simulink library "platooning_custom_blocks"  (R2018b)
settings: Solver=VariableStepAuto  StartTime=0.0  StopTime=10.0  RelTol=1e-3
undefined symbols (not defined in the file): AccPdl_pdlbpt, AccPdl_spdbpt, AccPdl_trqMap, adj_motEffMap, BETModel, BrkPdl_brkTrq, BrkPdl_pdlbpt, Cd_Map, Cd_Map_T2, CT_accPdl_pdlbpt, CT_accPdl_spdbpt, CT_accPdl_trqMap, CT_brkPdl_brkTrq, CT_brkPdl_pdlbpt, CTModel, d_11, d_22, DiscIntNeverNeededParam, init_veh_spd_mps, max_Cd_frac, min_Cd_frac, motSpdVec, motTrqVec, msk_init_pos_m, msk_mot_cont_trq, msk_mot_num, msk_mot_spd_bpt, N_OptResults, sim_t_step, simDrv, SPHETModel, t_step
libraries: simulink x19, $bdroot x16, dspstat3 x2, custom_func x1
(part 1 of 5)
settings Model: Creator=Aman-Home  LastModifiedBy=Aman-Home

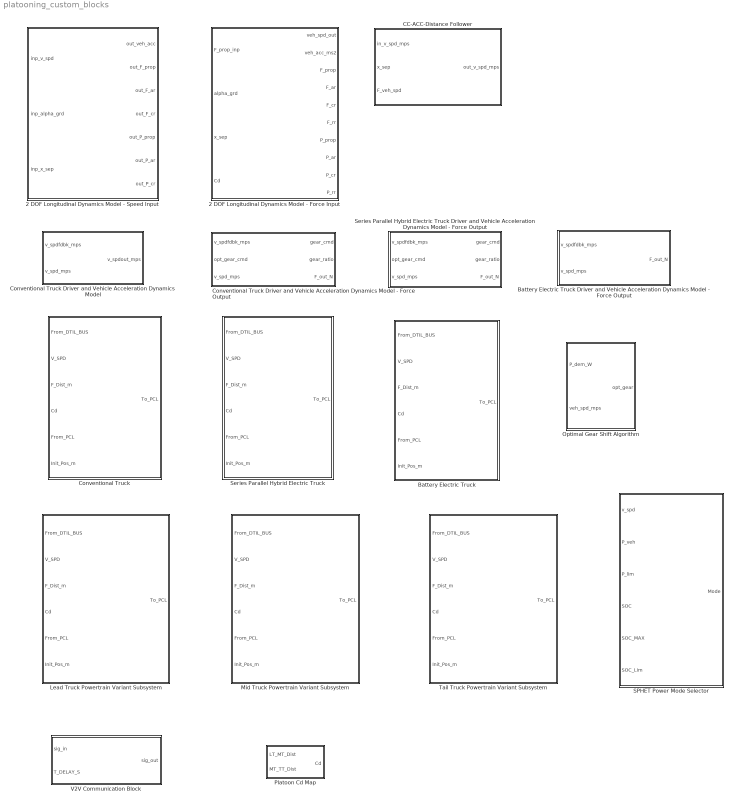
== system platooning_custom_blocks ==
  2 DOF Longitudinal Dynamics Model - Force Input : Subsystem  mask{msk_mass=CTModel.veh_mass_kg, msk_Af=CTModel.Af_m2, msk_Cd=CTModel.Cd_avg * ones([3 1]), msk_Cd_bpt=[5;10;15], msk_r_tire=CTModel.ld_tire_rad_m, msk_v_init=init_veh_spd_mps, msk_roadType=Smooth Concrete, msk_rho_air=1.227, msk_tstep=sim_t_step}
      mask prompts: msk_mass "Vehicle Mass [kg]:"; msk_Af "Vehicle Frontal Area [m^2]:"; msk_Cd "Vehicle Coefficient of Drag, Data Vector [n-by-1] (-):"; msk_Cd_bpt "Vehicle Coefficient of Drag, Breakpoint Vector [n-by-1] (meters):"; msk_r_tire "Vehicle Tire Radius [m]:"; msk_v_init "Vehicle Initial Speed [m/s]:"; msk_roadType "Road Type:"; msk_rho_air "Air density [kg/m^3]:"; msk_tstep "Simulation time step [s]:"
      mask init:
      | switch msk_roadType
      |     case 'Smooth Concrete'
      |         msk_roadType = 0;
      |     case 'Worn Concrete'
      |         msk_roadType = 1;
      |     case 'Hot Blacktop'
      |         msk_roadType = 2;
      | end
      mask TypeOptions msk_roadType: Smooth Concrete | Worn Concrete | Hot Blacktop
      mask DialogControl Container3 Prompt: Vehicle Parameters
      mask DialogControl Container6 Prompt: Road Parameters
      mask DialogControl Container7 Prompt: Environmental Parameters
      mask DialogControl Container9 Prompt: Simulation Parameters
  2 DOF Longitudinal Dynamics Model - Speed Input : Subsystem  mask{msk_mass=35380, msk_Af=4.5, msk_Cd=[0.3;0.2;0.1], msk_Cd_bpt=[5;10;15], msk_r_tire=0.5435, msk_roadType=Smooth Concrete, msk_rho_air=1.227, msk_tstep=t_step}
      mask prompts: msk_mass "Vehicle Mass [kg]:"; msk_Af "Vehicle Frontal Area [m^2]:"; msk_Cd "Vehicle Coefficient of Drag, Data Vector [n-by-1] (-):"; msk_Cd_bpt "Vehicle Coefficient of Drag, Breakpoint Vector [n-by-1] (meters):"; msk_r_tire "Vehicle Tire Radius [m]:"; msk_roadType "Road Type:"; msk_rho_air "Air density [kg/m^3]:"; msk_tstep "Simulation time step [s]:"
      mask init:
      | switch msk_roadType
      |     case 'Smooth Concrete'
      |         msk_roadType = 0;
      |     case 'Worn Concrete'
      |         msk_roadType = 1;
      |     case 'Hot Blacktop'
      |         msk_roadType = 2;
      | end
      mask TypeOptions msk_roadType: Smooth Concrete | Worn Concrete | Hot Blacktop
      mask DialogControl DescGroupVar Prompt: Description
      mask DialogControl DescTextVar Prompt: 2 DOF longitudinal vehicle dynamics model parameter settings.
      mask DialogControl Container3 Prompt: Vehicle Parameters
      mask DialogControl Container4 Prompt: Road Parameters
      mask DialogControl Container5 Prompt: Environment Parameters
      mask DialogControl Container6 Prompt: Simulation Parameters
  Battery Electric Truck : Subsystem  VariantControl=TT.Type == 3
  Battery Electric Truck Driver and Vehicle Acceleration Dynamics Model - Force Output : Subsystem  mask{msk_Kp=0.1, msk_Ki=0.001, msk_t_step=sim_t_step, msk_mtr_cont_trq=BETModel.cont_mtr_trq_map, msk_mtr_pk_trq=BETModel.peak_mtr_trq_map, msk_spd_bpt=BETModel.cont_mtr_trq_spdbpt, msk_gear_ratio=BETModel.gear_ratio, msk_num_motors=4, msk_acc_trqmap=AccPdl_trqMap, msk_acc_spdbpt=AccPdl_spdbpt, msk_acc_pdlbpt=AccPdl_pdlbpt, msk_brk_trq=BrkPdl_brkTrq, msk_brk_pdlbpt=BrkPdl_pdlbpt, msk_mass=BETModel.veh_mass_kg, msk_damp_acc=800, msk_damp_brk=0.1, msk_tire_radius=BETModel.ld_tire_rad_m, msk_brk_whl_num=10}
      mask prompts: msk_Kp "PI Control - Proportional Gain [Kp]:"; msk_Ki "PI Control - Integral Gain [Ki]:"; msk_t_step "Simulation time step [s]:"; msk_mtr_cont_trq "Motor Continuous Torque Vector []:"; msk_mtr_pk_trq "Motor Peak Torque Vector []:"; msk_spd_bpt "Motor Speed bpt []:"; msk_gear_ratio "Motor Gear Ratio []:"; msk_num_motors "Number of motors []:"; msk_acc_trqmap "Acceleration torque map:"; msk_acc_spdbpt "Acceleration torque map - speed breakpoint vector:"; msk_acc_pdlbpt "Acceleration torque map - pedal breakpoint vector:"; msk_brk_trq "Braking torque vector:"; msk_brk_pdlbpt "Braking torque - pedal breakpoint vector:"; msk_mass "Vehicle mass [kg]:"; msk_damp_acc "Vehicle system damping - acceleration [ms^-2]:"; msk_damp_brk "Vehicle system damping - braking [ms^-2]:"; msk_tire_radius "Vehicle tire radius [m]:"; msk_brk_whl_num "Number of Wheels with braking [-]:"
      mask DialogControl DescGroupVar Prompt: Driver Model Settings
      mask DialogControl DescTextVar Prompt: Enter parameters values and input data for the driver model.
      mask DialogControl Container3 Prompt: Motor Parameters
      mask DialogControl Container4 Prompt: Pedal Maps
      mask DialogControl Container5 Prompt: Vehicle Parameters
  CC-ACC-Distance Follower : Subsystem  mask{msk_cc_mode=Disabled, msk_cc_setspd=25, msk_cc_time=100, msk_ACC_Kp=0.5, msk_ACC_Ki=0.01, msk_ACC_Kd=0, msk_ACC_setdist_init=70, msk_platoon_time=200, msk_ACC_setdist_final=15}
      mask prompts: msk_cc_mode "Select the controller mode:"; msk_cc_setspd "Cruise Control Set Speed:"; msk_cc_time "Cruise Control Activation Time [s]:"; msk_ACC_Kp "ACC - Distance Control, Kp:"; msk_ACC_Ki "ACC - Distance Control, Ki:"; msk_ACC_Kd "ACC - Distance Control, Kd:"; msk_ACC_setdist_init "ACC - Pre-Platoon Distance Setting [m]:"; msk_platoon_time "ACC - Platooning Start Time [s]:"; msk_ACC_setdist_final "ACC - Platoon Distance Setting [m]:"
      mask init:
      | switch msk_cc_mode
      |     case 'Disabled'
      |         msk_cc_mode = 0;
      |     case 'Activate - Cruise Control'
      |         msk_cc_mode = 1;
      |     case 'Activate - Adaptive Cruise Control'
      |         msk_cc_mode = 2;
      |     case 'Activate - Distance Following'
      |         msk_cc_mode = 3;
      | end
      mask TypeOptions msk_cc_mode: Disabled | Activate - Cruise Control | Activate - Adaptive Cruise Control | Activate - Distance Following
      mask Callback msk_cc_mode:
      | % Get the mask parameter values. This is a cell
      | %   array of character vectors.
      | maskStr = get_param(gcb,'msk_cc_mode');
      | 
      | % The pop-up menu is the first mask parameter.
      | %   Check the value selected in the pop-up
      | if strcmp(maskStr(1),'A') && strcmp(maskStr(12),'C')    % Activated - Cruise Control
      | 
      |     % Set the visibility of both parameters on when
      |     %   User-defined is selected in the pop-up.
      |     set_param(gcb,'MaskVisibilities',{'on';'on';'on';'off';'off';'off';'off';'off';'off'})
      | 
      | elseif strcmp(maskStr(1),'A') && strcmp(maskStr(12),'A')    % Activated - Adaptive Cruise Control
      | 
      |     % Turn off the visibility of the Value field
      |     %   when User-defined is not selected.
      | 
      |     set_param(gcb,'MaskVisibilities',{'on';'on';'on';'on';'on';'on';'on';'on';'on'})
      | 
      | elseif strcmp(maskStr(1),'A') && strcmp(maskStr(12),'D')    % Activated - Distance Following
      | 
      |     set_param(gcb,'MaskVisibilities',{'on';'on';'on';'on';'on';'on';'on';'on';'on'})
      | 
      | else
      | 
      |      set_param(gcb,'MaskVisibilities',{'on';'off';'off';'off';'off';'off';'off';'off';'off'})
      | 
      |     % Set the character vector in the Values field equal to the
      |     % character vector selected in the Gain pop-up menu.
      | 
      |     %maskStr{2}=maskStr{1};
      |     %set_param(gcb,'t_shutfault',inf);
      | end
      mask DialogControl DescGroupVar Prompt: Autonomous Speed Controller
      mask DialogControl DescTextVar Prompt: This block is used to enable and disable Cruise Control (CC), Adaptive Cruise Control (ACC) and Distance Following (DF) algorithms.
  Conventional Truck : Subsystem  VariantControl=LT.Type == 1
  Conventional Truck Driver and Vehicle Acceleration Dynamics Model : Subsystem  mask{msk_Kp=0.0075, msk_Ki=0.005, msk_t_step=t_step, msk_gear_ratio_vec=[14.43,11.05,8.44,6.46,4.95,3.79,2.91,2.23,1.70], msk_gearShft_UL=[3, 5, 10, 14, 18, 22, 26, 32, 45], msk_gearShft_LL=[0, 2, 4, 8, 12, 16, 20, 24, 30], msk_gearInit=1, msk_acc_trqmap=CT_accPdl_trqMap, msk_acc_spdbpt=CT_accPdl_spdbpt, msk_acc_pdlbpt=CT_accPdl_pdlbpt, msk_brk_trq=CT_brkPdl_brkTrq, msk_brk_pdlbpt=CT_brkPdl_pdlbpt, msk_mass=35000, msk_damp_acc=800, msk_damp_brk=0.1, msk_fd_ratio=2.8, msk_tire_radius=0.5456, msk_max_trq=2100, msk_brk_whl_num=10}
      mask prompts: msk_Kp "PI Control - Proportional Gain [Kp]:"; msk_Ki "PI Control - Integral Gain [Ki]:"; msk_t_step "Simulation time step [s]:"; msk_gear_ratio_vec "Gear ratio vector []:"; msk_gearShft_UL "Gear shift speed - Upper Limit vector []:"; msk_gearShft_LL "Gear shift speed - Lower Limit vector []:"; msk_gearInit "Initial Gear (non-zero):"; msk_acc_trqmap "Acceleration torque map:"; msk_acc_spdbpt "Acceleration torque map - speed breakpoint vector:"; msk_acc_pdlbpt "Acceleration torque map - pedal breakpoint vector:"; msk_brk_trq "Braking torque vector:"; msk_brk_pdlbpt "Braking torque - pedal breakpoint vector:"; msk_mass "Vehicle mass [kg]:"; msk_damp_acc "Vehicle system damping - acceleration [ms^-2]:"; msk_damp_brk "Vehicle system damping - braking [ms^-2]:"; msk_fd_ratio "Vehicle final drive ratio []:"; msk_tire_radius "Vehicle tire radius [m]:"; msk_max_trq "Maximum Engine Torque [Nm]:"; msk_brk_whl_num "Number of Wheels with braking [-]:"
      mask DialogControl DescGroupVar Prompt: Driver Model Settings
      mask DialogControl DescTextVar Prompt: Enter parameters values and input data for the driver model.
      mask DialogControl Container3 Prompt: Gear Shift Parameters
      mask DialogControl Container4 Prompt: Pedal Maps
      mask DialogControl Container5 Prompt: Vehicle Parameters
  Conventional Truck Driver and Vehicle Acceleration Dynamics Model - Force Output : Subsystem  mask{msk_Kp=0.1, msk_Ki=0.001, msk_t_step=sim_t_step, msk_gear_ratio_vec=CTModel.gear_ratios, msk_gearShft_UL=[3, 5, 9, 13, 17, 21, 25, 29, 33, 45], msk_gearShft_LL=[0, 2, 4, 8, 12, 16, 20, 24, 28, 32], msk_gearInit=1, msk_acc_trqmap=AccPdl_trqMap, msk_acc_spdbpt=AccPdl_spdbpt, msk_acc_pdlbpt=AccPdl_pdlbpt, msk_brk_trq=BrkPdl_brkTrq, msk_brk_pdlbpt=BrkPdl_pdlbpt, msk_mass=CTModel.veh_mass_kg, msk_damp_acc=800, msk_damp_brk=0.1, msk_fd_ratio=CTModel.fd_ratio, msk_tire_radius=CTModel.ld_tire_rad_m, msk_max_trq=max(CTModel.peak_eng_trq_map), msk_brk_whl_num=10}
      mask prompts: msk_Kp "PI Control - Proportional Gain [Kp]:"; msk_Ki "PI Control - Integral Gain [Ki]:"; msk_t_step "Simulation time step [s]:"; msk_gear_ratio_vec "Gear ratio vector []:"; msk_gearShft_UL "Gear shift speed - Upper Limit vector []:"; msk_gearShft_LL "Gear shift speed - Lower Limit vector []:"; msk_gearInit "Initial Gear (non-zero):"; msk_acc_trqmap "Acceleration torque map:"; msk_acc_spdbpt "Acceleration torque map - speed breakpoint vector:"; msk_acc_pdlbpt "Acceleration torque map - pedal breakpoint vector:"; msk_brk_trq "Braking torque vector:"; msk_brk_pdlbpt "Braking torque - pedal breakpoint vector:"; msk_mass "Vehicle mass [kg]:"; msk_damp_acc "Vehicle system damping - acceleration [ms^-2]:"; msk_damp_brk "Vehicle system damping - braking [ms^-2]:"; msk_fd_ratio "Vehicle final drive ratio []:"; msk_tire_radius "Vehicle tire radius [m]:"; msk_max_trq "Maximum Engine Torque [Nm]:"; msk_brk_whl_num "Number of Wheels with braking [-]:"
      mask DialogControl DescGroupVar Prompt: Driver Model Settings
      mask DialogControl DescTextVar Prompt: Enter parameters values and input data for the driver model.
      mask DialogControl Container3 Prompt: Gear Shift Parameters
      mask DialogControl Container4 Prompt: Pedal Maps
      mask DialogControl Container5 Prompt: Vehicle Parameters
  Lead Truck Powertrain Variant Subsystem : Subsystem  Variant=on
  Mid Truck Powertrain Variant Subsystem : Subsystem  Variant=on
  Optimal Gear Shift Algorithm : Subsystem  mask{msk_tire_radius_m=CTModel.ld_tire_rad_m, msk_trns_eff_avg=mean(CTModel.gear_eff), msk_init_gear=1}
      mask prompts: msk_tire_radius_m "Vehicle tire radius :"; msk_trns_eff_avg "Average transmission efficiency :"; msk_init_gear "Initial gear selection :"
      mask DialogControl DescGroupVar Prompt: Optimal Gear Shift Algorithm
      mask DialogControl DescTextVar Prompt: The block computes optimal gear based on the power demand and vehicle speed by minimizing fuel consumption.
  Platoon Cd Map : Subsystem  mask{msk_platoon_type=Individual, pos=Lead, msk_platoon_cd_map=Cd_Map, msk_platoon_cd_map_t2=Cd_Map_T2, msk_d1_bpt=d_11, msk_d2_bpt=d_22, msk_cd_avg=0.52}
      mask prompts: msk_platoon_type "Platoon Type"; pos "Platoon Position"; msk_platoon_cd_map "Platoon Cd Map, 3 Truck [m-n-3]:"; msk_platoon_cd_map_t2 "Platoon Cd Map. 2 Truck [m-2]:"; msk_d1_bpt "LT-MT Distance Breakpoint [m]:"; msk_d2_bpt "MT-TT Distance Breakpoint [m]:"; msk_cd_avg "Average Cd [-]:"
      mask init:
      | switch pos
      |     case 'Lead'
      |         pos = 1;
      |     case 'Middle'
      |         pos = 2;
      |     case 'Tail'
      |         pos = 3;
      | end
      | switch msk_platoon_type
      |     case 'Individual'
      |         msk_platoon_type = 1;
      |     case 'Two Truck'
      |         msk_platoon_type = 2;
      |     case 'Three Truck'
      |         msk_platoon_type = 3;
      | end
      mask TypeOptions msk_platoon_type: Individual | Two Truck | Three Truck
      mask TypeOptions pos: Lead | Middle | Tail
      mask DialogControl ParameterGroupVar Prompt: Truck Position Selector
      mask DialogControl Container3 Prompt: Drag Coefficient Map
  SPHET Power Mode Selector : Stateflow chart  TreatAsAtomicUnit=on
  Series Parallel Hybrid Electric Truck : Subsystem  VariantControl=MT.Type == 2
  Series Parallel Hybrid Electric Truck Driver and Vehicle Acceleration Dynamics Model - Force Output : Subsystem  mask{msk_mass=SPHETModel.veh_mass_kg, msk_damp_acc=800, msk_damp_brk=0.1, msk_tire_radius=SPHETModel.ld_tire_rad_m, msk_brk_whl_num=10, msk_fd_ratio=SPHETModel.fd_ratio, msk_Kp=0.1, msk_Ki=0.001, msk_t_step=sim_t_step, msk_eng_pk_trq=SPHETModel.peak_eng_trq_map, msk_eng_spd_bpt=SPHETModel.peak_eng_trq_spd_bpt, msk_gear_ratio_vec=SPHETModel.gear_ratios, msk_gearInit=1, msk_gearShft_UL=[3, 5, 9, 13, 17, 21, 25, 29, 33, 45], msk_gearShft_LL=[0, 2, 4, 8, 12, 16, 20, 24, 28, 32], msk_plnt_c_r_ratio=SPHETModel.mg_ratio_eng_out, msk_plnt_m_r_ratio=SPHETModel.mg_ratio_mot_out, msk_plnt_s_r_ratio=1/SPHETModel.mg_ratio_out_gen, msk_plnt_s_c_ratio=1/SPHETModel.mg_ratio_eng_gen, msk_mtr_cont_trq=SPHETModel.cont_mtr_trq_map, msk_mtr_pk_trq=SPHETModel.peak_mtr_trq_map, msk_spd_bpt=SPHETModel.cont_mtr_trq_spdbpt, msk_gear_ratio=SPHETModel.mg_ratio_mot_out, msk_num_motors=1, msk_acc_trqmap=AccPdl_trqMap, msk_acc_spdbpt=AccPdl_spdbpt, msk_acc_pdlbpt=AccPdl_pdlbpt, msk_brk_trq=BrkPdl_brkTrq, msk_brk_pdlbpt=BrkPdl_pdlbpt}
      mask prompts: msk_mass "Vehicle mass [kg]:"; msk_damp_acc "Vehicle system damping - acceleration [ms^-2]:"; msk_damp_brk "Vehicle system damping - braking [ms^-2]:"; msk_tire_radius "Vehicle tire radius [m]:"; msk_brk_whl_num "Number of Wheels with braking [-]:"; msk_fd_ratio "Final drive ratio [-]:"; msk_Kp "PI Control - Proportional Gain [Kp]:"; msk_Ki "PI Control - Integral Gain [Ki]:"; msk_t_step "Simulation time step [s]:"; msk_eng_pk_trq "Engine peak torque, propulsion [Nm] :"; msk_eng_spd_bpt "Engine speed breakpoint [RPM]"; msk_gear_ratio_vec "Gear ratio vector []:"; msk_gearInit "Initial gear number :"; msk_gearShft_UL "Gear shift, upper speed limit vector []:"; msk_gearShft_LL "Gear shift, lower speed limit vector []:"; msk_plnt_c_r_ratio "Engine to Output (C to R ratio) :"; msk_plnt_m_r_ratio "Motor to Output (M to R ratio) :"; msk_plnt_s_r_ratio "Generator to Output (S to R ratio) :"; msk_plnt_s_c_ratio "Generator to Engine (S to C ratio) :"; msk_mtr_cont_trq "Motor Continuous Torque Vector []:"; msk_mtr_pk_trq "Motor Peak Torque Vector []:"; msk_spd_bpt "Motor Speed bpt []:"; msk_gear_ratio "Motor Gear Ratio []:"; msk_num_motors "Number of motors []:"; msk_acc_trqmap "Acceleration torque map:"; msk_acc_spdbpt "Acceleration torque map - speed breakpoint vector:"; msk_acc_pdlbpt "Acceleration torque map - pedal breakpoint vector:"; msk_brk_trq "Braking torque vector:"; msk_brk_pdlbpt "Braking torque - pedal breakpoint vector:"
      mask DialogControl DescGroupVar Prompt: Driver Model Settings
      mask DialogControl DescTextVar Prompt: Enter parameters values and input data for the driver model.
      mask DialogControl Container14 Prompt: Vehicle Parameters
      mask DialogControl Container7 Prompt: Simulation/Control Parameters
      mask DialogControl Container8 Prompt: Engine Parameters
      mask DialogControl Container11 Prompt: Transmission Parameters
      mask DialogControl Container16 Prompt: Planetary Gearbox Parameters
      mask DialogControl Container12 Prompt: Motor Parameters
      mask DialogControl Container13 Prompt: Pedal Maps
  Tail Truck Powertrain Variant Subsystem : Subsystem  Variant=on
  V2V Communication Block : Subsystem  mask{msk_t_step_s=0.01, msk_snr_value=20}
      mask prompts: msk_t_step_s "Simulation time step [s] :"; msk_snr_value "Signal-to-Noise ratio [-] :"

== system platooning_custom_blocks/2 DOF Longitudinal Dynamics Model - Force Input ==
  F_prop_inp : Inport
  alpha_grd : Inport  Port=2
  x_sep : Inport  Port=3
  Cd : Inport  Port=4
  2 DOF Longitudinal Dynamics Model - Force Input : MATLAB Function  TreatAsAtomicUnit=on
  Constant2 : Constant  Value=msk_tstep
  Constant3 : Constant  Value=msk_mass
  Constant4 : Constant  Value=msk_rho_air
  Constant5 : Constant  Value=msk_Af
  Constant6 : Constant  Value=msk_r_tire
  Constant7 : Constant  Value=msk_roadType
  Constant8 : Constant  Value=msk_v_init
  Rate Transition : RateTransition  OutPortSampleTime=sim_t_step
  Rate Transition1 : RateTransition  OutPortSampleTime=sim_t_step
  Rate Transition2 : RateTransition  OutPortSampleTime=sim_t_step
  veh_spd_out : Outport
  veh_acc_ms2 : Outport  Port=2
  F_prop : Outport  Port=3
  F_ar : Outport  Port=4
  F_cr : Outport  Port=5
  F_rr : Outport  Port=6
  P_prop : Outport  Port=7
  P_ar : Outport  Port=8
  P_cr : Outport  Port=9
  P_rr : Outport  Port=10
  wires:
  Cd/1 -> 2 DOF Longitudinal Dynamics Model - Force Input/9(msk_Cd)
  Rate Transition2/1 -> 2 DOF Longitudinal Dynamics Model - Force Input/3(x_sep)
  Rate Transition1/1 -> 2 DOF Longitudinal Dynamics Model - Force Input/2(alpha_grd)
  Rate Transition/1 -> 2 DOF Longitudinal Dynamics Model - Force Input/1("F_prop ")
  2 DOF Longitudinal Dynamics Model - Force Input/10(P_rr) -> P_rr/1
  2 DOF Longitudinal Dynamics Model - Force Input/6(F_rr) -> F_rr/1
  2 DOF Longitudinal Dynamics Model - Force Input/1(veh_spd_out) -> veh_spd_out/1
  Constant7/1 -> 2 DOF Longitudinal Dynamics Model - Force Input/11(msk_roadType)
  2 DOF Longitudinal Dynamics Model - Force Input/5(F_cr) -> F_cr/1
  Constant4/1 -> 2 DOF Longitudinal Dynamics Model - Force Input/7(msk_rho_air)
  Constant8/1 -> 2 DOF Longitudinal Dynamics Model - Force Input/4(v_init)
  Constant5/1 -> 2 DOF Longitudinal Dynamics Model - Force Input/8(msk_Af)
  x_sep/1 -> Rate Transition2/1
  Constant2/1 -> 2 DOF Longitudinal Dynamics Model - Force Input/5(msk_tstep)
  Constant3/1 -> 2 DOF Longitudinal Dynamics Model - Force Input/6(msk_mass)
  alpha_grd/1 -> Rate Transition1/1
  Constant6/1 -> 2 DOF Longitudinal Dynamics Model - Force Input/10(msk_r_tire)
  2 DOF Longitudinal Dynamics Model - Force Input/3(F_prop) -> F_prop/1
  2 DOF Longitudinal Dynamics Model - Force Input/2(veh_acc_ms2) -> veh_acc_ms2/1
  2 DOF Longitudinal Dynamics Model - Force Input/7(P_prop) -> P_prop/1
  2 DOF Longitudinal Dynamics Model - Force Input/9(P_cr) -> P_cr/1
  2 DOF Longitudinal Dynamics Model - Force Input/4(F_ar) -> F_ar/1
  2 DOF Longitudinal Dynamics Model - Force Input/8(P_ar) -> P_ar/1
  F_prop_inp/1 -> Rate Transition/1

== system platooning_custom_blocks/2 DOF Longitudinal Dynamics Model - Speed Input ==
  inp_v_spd : Inport
  inp_alpha_grd : Inport  Port=2
  inp_x_sep : Inport  Port=3
  2DOF Longitudinal Dynamics Model - Speed Input : MATLAB Function  TreatAsAtomicUnit=on
  Cd_v_xsep : Lookup_n-D  NumberOfTableDimensions=1  BreakpointsForDimension1=msk_Cd_bpt  Table=msk_Cd  InternalRulePriority=Speed  RndMeth=Simplest  InputSameDT=on
  Constant : Constant  Value=msk_tstep
  Constant1 : Constant  Value=msk_mass
  Constant2 : Constant  Value=msk_rho_air
  Constant3 : Constant  Value=msk_Af
  Constant5 : Constant  Value=msk_r_tire
  Constant6 : Constant  Value=msk_roadType
  out_veh_acc : Outport
  out_F_prop : Outport  Port=2
  out_F_ar : Outport  Port=3
  out_F_cr : Outport  Port=4
  out_P_prop : Outport  Port=5
  out_P_ar : Outport  Port=6
  out_P_cr : Outport  Port=7
  wires:
  2DOF Longitudinal Dynamics Model - Speed Input/1(veh_acc_ms2) -> out_veh_acc/1
  Constant5/1 -> 2DOF Longitudinal Dynamics Model - Speed Input/9(msk_r_tire)
  inp_v_spd/1 -> 2DOF Longitudinal Dynamics Model - Speed Input/1(v_spd)
  2DOF Longitudinal Dynamics Model - Speed Input/2(F_prop) -> out_F_prop/1
  2DOF Longitudinal Dynamics Model - Speed Input/3(F_ar) -> out_F_ar/1
  2DOF Longitudinal Dynamics Model - Speed Input/4(F_cr) -> out_F_cr/1
  inp_alpha_grd/1 -> 2DOF Longitudinal Dynamics Model - Speed Input/2(alpha_grd)
  Constant/1 -> 2DOF Longitudinal Dynamics Model - Speed Input/4(msk_tstep)
  Constant2/1 -> 2DOF Longitudinal Dynamics Model - Speed Input/6(msk_rho_air)
  Constant3/1 -> 2DOF Longitudinal Dynamics Model - Speed Input/7(msk_Af)
  Constant6/1 -> 2DOF Longitudinal Dynamics Model - Speed Input/10(msk_roadType)
  Constant1/1 -> 2DOF Longitudinal Dynamics Model - Speed Input/5(msk_mass)
  inp_x_sep/1 -> Cd_v_xsep/1, 2DOF Longitudinal Dynamics Model - Speed Input/3(x_sep)
  2DOF Longitudinal Dynamics Model - Speed Input/6(P_ar) -> out_P_ar/1
  2DOF Longitudinal Dynamics Model - Speed Input/5(P_prop) -> out_P_prop/1
  2DOF Longitudinal Dynamics Model - Speed Input/7(P_cr) -> out_P_cr/1
  Cd_v_xsep/1 -> 2DOF Longitudinal Dynamics Model - Speed Input/8(msk_Cd)

== system platooning_custom_blocks/Battery Electric Truck ==
  From_DTIL_BUS : Inport
  V_SPD : Inport  Port=2
  F_Dist_m : Inport  Port=3
  Cd : Inport  Port=4
  From_PCL : Inport  Port=5
  Init_Pos_m : Inport  Port=6
  2 DOF Longitudinal Dynamics Model - Force Input : $bdroot/2 DOF Longitudinal Dynamics Model - Force Input  msk_mass=BETModel.veh_mass_kg  msk_Af=BETModel.Af_m2  msk_Cd=BETModel.Cd_avg * ones([3 1])  msk_Cd_bpt=[5;10;15]  msk_r_tire=BETModel.ld_tire_rad_m  msk_v_init=init_veh_spd_mps  msk_roadType=Smooth Concrete  msk_rho_air=1.227  msk_tstep=sim_t_step
  Battery Electric Post-Processing : Subsystem  mask{msk_cell_Q_Ah=BETModel.Q_cell_max_Ah, msk_cell_Vnom=BETModel.V_cell_nom, msk_batt_Ns=BETModel.Ns, msk_batt_Np=BETModel.Np, msk_batt_Nmod=BETModel.Nmod, msk_batt_soc_init=1, msk_distwin=1000}
      mask prompts: msk_cell_Q_Ah "Battery cell capacity, Q [Ah]:"; msk_cell_Vnom "Battery cell nominal voltage, Vnom [V]:"; msk_batt_Ns "Number of cells in series, Ns [-]:"; msk_batt_Np "Number of cells in parallel, Np [-]:"; msk_batt_Nmod "Number of modules, Nmod [-]:"; msk_batt_soc_init "Battery initial SOC, SOCinit/100 :"; msk_distwin "Short term averaging, distance window [m]:"
      mask DialogControl DescGroupVar Prompt: Post-Processing Block - Battery Electric Vehicle
      mask DialogControl DescTextVar Prompt: This block computes overall energy consumption and distance-to-empty for a battery electric vehicle.
  Battery Electric Powertrain Power Loss Model : Subsystem  mask{msk_mot_eff=BETModel.mtr_eff, msk_gear_eff=BETModel.gear_eff, msk_mot_gbx_rat=BETModel.gear_ratio, msk_tire_radius_m=BETModel.ld_tire_rad_m, msk_t_step=sim_t_step, msk_cell_Q_Ah=BETModel.Q_cell_max_Ah, msk_cell_Vnom=BETModel.V_cell_nom, msk_batt_Ns=BETModel.Ns, msk_batt_Np=BETModel.Np, msk_batt_Nmod=BETModel.Nmod, msk_batt_soc_init=1, msk_dchglim10s=BETModel.DchgCurrLim_10sAvg_A, msk_cellTempbpt=BETModel.cellTempbpt_C, msk_soc_bpt=BETModel.socbpt, msk_batt_R0=BETModel.batt_R0, msk_batt_R1=BETModel.batt_R1, msk_batt_R2=BETModel.batt_R2, msk_batt_C1=BETModel.batt_C1, msk_batt_C2=BETModel.batt_C2, msk_batt_soc_bpt=BETModel.batt_socbpt, msk_P_aux_mech_load=BETModel.P_aux_mech, msk_P_aux_elec_load=BETModel.P_aux_elec, msk_P_aux_load_frac=BETModel.P_aux_load_frac, msk_snr_P_aux=25}
      mask prompts: msk_mot_eff "Motor efficiency/100 [-]:"; msk_gear_eff "Gearbox efficiency/100 [-]:"; msk_mot_gbx_rat "Gearbox ratio, n:1 [-]:"; msk_tire_radius_m "Loaded tire radius [m]:"; msk_t_step "Simulation time step [s]:"; msk_cell_Q_Ah "Battery cell capacity, Q [Ah]:"; msk_cell_Vnom "Battery cell nominal voltage, Vnom [V]:"; msk_batt_Ns "Number of cells in series, Ns [-]:"; msk_batt_Np "Number of cells in parallel, Np [-]:"; msk_batt_Nmod "Number of battery modules, Nmod [-]:"; msk_batt_soc_init "Battery initial SOC [SOC/100]:"; msk_dchglim10s "Battery 10s Discharge Limit []:"; msk_cellTempbpt "Battery cell temperature breakpoint []:"; msk_soc_bpt "Battery SOC breakpoint []:"; msk_batt_R0 "Battery Resistance R0 LUT []:"; msk_batt_R1 "Battery Resistance R1 LUT []:"; msk_batt_R2 "Battery Resistance R2 LUT []:"; msk_batt_C1 "Battery Capacitance C1 LUT []:"; msk_batt_C2 "Battery Capacitance C2 LUT []:"; msk_batt_soc_bpt "Battery internal params SOC breakpoints []:"; msk_P_aux_mech_load "Auxiliary load power, mechanical [W]:"; msk_P_aux_elec_load "Auxiliary load power, electrical [W]:"; msk_P_aux_load_frac "Auxiliary load fraction [-]:"; msk_snr_P_aux "Signal-to-Noise ratio [-]:"
      mask DialogControl DescGroupVar Prompt: Battery Electric Powertrain Mode
      mask DialogControl DescTextVar Prompt: Parameter settings for systems and components in the Battery Electric Powertrain
      mask DialogControl Container7 Prompt: Drivetrain Parameters
      mask DialogControl Container9 Prompt: Simulation Parameters
      mask DialogControl Container10 Prompt: Battery Parameters
      mask DialogControl Container4 Prompt: Internal Battery Parameters
      mask DialogControl Container11 Prompt: Auxiliary Load Parameters
  Battery Electric Truck Energy Management System : Subsystem  mask{msk_cont_chg_map=BETModel.ChgCurrLim_cont_A, msk_soc_bpt=BETModel.socbpt, msk_cell_temp_bpt=BETModel.cellTempbpt_C, msk_mtr_eff=BETModel.mtr_eff * BETModel.gear_eff, msk_num_mtr=4}
      mask prompts: msk_cont_chg_map "Battery continuous charge current map []:"; msk_soc_bpt "Battery SOC breakpoint []:"; msk_cell_temp_bpt "Battery Temperature breakpoint []:"; msk_mtr_eff "Motor efficiency/100 :"; msk_num_mtr "Number of motors :"
      mask DialogControl DescGroupVar Prompt: Battery Electric Energy Management System
      mask DialogControl DescTextVar Prompt: Parameter settings for the Battery Electric Energy Management Systems
  Battery Electric Truck Driver and Vehicle Acceleration Dynamics Model - Force Output : $bdroot/Battery Electric Truck Driver and  Vehicle Acceleration Dynamics Model  - Force Output  msk_Kp=0.1  msk_Ki=0.001  msk_t_step=sim_t_step  msk_mtr_cont_trq=BETModel.cont_mtr_trq_map  msk_mtr_pk_trq=BETModel.peak_mtr_trq_map  msk_spd_bpt=BETModel.cont_mtr_trq_spdbpt  msk_gear_ratio=BETModel.gear_ratio  msk_num_motors=2  msk_acc_trqmap=AccPdl_trqMap  msk_acc_spdbpt=AccPdl_spdbpt  msk_acc_pdlbpt=AccPdl_pdlbpt  msk_brk_trq=BrkPdl_brkTrq  msk_brk_pdlbpt=BrkPdl_pdlbpt  msk_mass=BETModel.veh_mass_kg  msk_damp_acc=800  msk_damp_brk=0.1  msk_tire_radius=BETModel.ld_tire_rad_m  msk_brk_whl_num=18
  Bus Creator1 : BusCreator  Inputs=2
  Bus Creator2 : BusCreator  Inputs=4
  Bus Creator3 : BusCreator  Inputs=4
  Bus Selector2 : BusSelector  OutputSignals=tail_grade_pct
  Bus Selector3 : BusSelector  OutputSignals=clock
  Rate Transition : RateTransition  OutPortSampleTime=sim_t_step
  Rate Transition1 : RateTransition  OutPortSampleTime=sim_t_step
  Rate Transition2 : RateTransition  OutPortSampleTime=sim_t_step
  Terminator : Terminator
  To_PCL : Outport
  wires:
  Cd/1 -> 2 DOF Longitudinal Dynamics Model - Force Input/4
  Init_Pos_m/1 -> Battery Electric Powertrain Power Loss Model/5(Init_Pos_m)
  Rate Transition2/1 -> 2 DOF Longitudinal Dynamics Model - Force Input/3
  Rate Transition1/1 -> 2 DOF Longitudinal Dynamics Model - Force Input/2
  Rate Transition/1 -> 2 DOF Longitudinal Dynamics Model - Force Input/1
  Battery Electric Truck Energy Management System/1(EMC_to_PropSys) -> Battery Electric Powertrain Power Loss Model/4(EM_control_bus)
  From_PCL/1 -> Battery Electric Truck Energy Management System/2(From_PCL_BUS)
  2 DOF Longitudinal Dynamics Model - Force Input/4 -> Bus Creator2/2  "F_ar"
  Battery Electric Post-Processing/1(To_PCL_BUS) -> To_PCL/1
  Bus Creator3/1 -> Battery Electric Powertrain Power Loss Model/2(Power_data_bus)  "PowerDatBus"
  Bus Selector3/1 -> Battery Electric Powertrain Power Loss Model/3(clock)  "<clock>"
  2 DOF Longitudinal Dynamics Model - Force Input/9 -> Bus Creator3/3  "P_cr"
  From_DTIL_BUS/1 -> Bus Selector3/1, Bus Selector2/1
  2 DOF Longitudinal Dynamics Model - Force Input/5 -> Bus Creator2/3  "F_cr"
  V_SPD/1 -> Battery Electric Truck Driver and Vehicle Acceleration Dynamics Model - Force Output/2
  2 DOF Longitudinal Dynamics Model - Force Input/2 -> Bus Creator1/2  "vehAccOut"
  Bus Creator1/1 -> Battery Electric Powertrain Power Loss Model/1(Motion_data_bus)  "MotionDatBus"
  2 DOF Longitudinal Dynamics Model - Force Input/8 -> Bus Creator3/2  "P_ar"
  2 DOF Longitudinal Dynamics Model - Force Input/10 -> Bus Creator3/4  "P_rr"
  2 DOF Longitudinal Dynamics Model - Force Input/7 -> Bus Creator3/1  "P_prop"
  Bus Creator2/1 -> Terminator/1
  Battery Electric Truck Driver and Vehicle Acceleration Dynamics Model - Force Output/1 -> Rate Transition/1  "F_cmd_out"
  2 DOF Longitudinal Dynamics Model - Force Input/1 -> Bus Creator1/1, Battery Electric Truck Driver and Vehicle Acceleration Dynamics Model - Force Output/1  "vehSpdOut"
  F_Dist_m/1 -> Rate Transition2/1
  2 DOF Longitudinal Dynamics Model - Force Input/6 -> Bus Creator2/4  "F_rr"
  2 DOF Longitudinal Dynamics Model - Force Input/3 -> Bus Creator2/1  "F_prop"
  Bus Selector2/1 -> Rate Transition1/1  "<tail_grade_pct>"
  Battery Electric Powertrain Power Loss Model/1(PropSys_to_EMC) -> Battery Electric Post-Processing/1(PropSys_to_EMC), Battery Electric Truck Energy Management System/1(PropSys_to_EMC)

== system platooning_custom_blocks/Battery Electric Truck Driver and Vehicle Acceleration Dynamics Model - Force Output ==
  note: Peak torque map can be added with a timer control
  v_spdfdbk_mps : Inport
  v_spd_mps : Inport  Port=2
  Acc_Pedal : Saturate  UpperLimit=1  LowerLimit=0
  Acceleration Torque LUT : Lookup_n-D  BreakpointsForDimension1=msk_acc_spdbpt  BreakpointsForDimension2=msk_acc_pdlbpt  Table=msk_acc_trqmap  InternalRulePriority=Speed  RndMeth=Simplest  InputSameDT=on
  Add : Sum  Inputs=-+|
  Braking Torque LUT : Lookup_n-D  NumberOfTableDimensions=1  BreakpointsForDimension1=msk_brk_pdlbpt  Table=msk_brk_trq * -1  InternalRulePriority=Speed  RndMeth=Simplest  InputSameDT=on
  Braking Wheels : Gain  Gain=msk_brk_whl_num
  Brk_Pedal : Saturate  UpperLimit=0  LowerLimit=-1
  Constant : Constant  Value=msk_gear_ratio
  Constant1 : Constant  Value=1/msk_tire_radius
  Constant2 : Constant  Value=msk_num_motors
  Gain : Gain  Gain=-1
  Motor Continuous Torque LUT : Lookup_n-D  NumberOfTableDimensions=1  BreakpointsForDimension1=msk_spd_bpt  Table=msk_mtr_cont_trq  InternalRulePriority=Speed  RndMeth=Simplest  InputSameDT=on
  PID Controller : simulink/Continuous/PID Controller  Controller=PI  Form=Parallel  TimeDomain=Continuous-time  SampleTime=-1  IntegratorMethod=Forward Euler  FilterMethod=Forward Euler  ControllerParametersSource=internal  P=msk_Kp  I=msk_Ki  D=0  UseFilter=on  N=100  TunerSelectOption=Transfer Function Based (PID Tuner App)  InitialConditionSource=internal  InitialConditionForIntegrator=0  InitialConditionForFilter=0  DifferentiatorICPrevScaledInput=0  ExternalReset=none  TrackingMode=off  Kt=1  LimitOutput=on  UpperSaturationLimit=1  LowerSaturationLimit=-1  LinearizeAsGain=on  AntiWindupMode=clamping  Kb=1  POutMin=[]  POutMax=[]  IOutMin=[]  IOutMax=[]  DOutMin=[]  DOutMax=[]  NOutMin=[]  NOutMax=[]  SumOutMin=[]  SumOutMax=[]  SaturationOutMin=[]  SaturationOutMax=[]  PParamMin=[]  PParamMax=[]  IParamMin=[]  IParamMax=[]  DParamMin=[]  DParamMax=[]  NParamMin=[]  NParamMax=[]  KbParamMin=[]  KbParamMax=[]  KtParamMin=[]  KtParamMax=[]  KbOutMin=[]  KbOutMax=[]  KtOutMin=[]  KtOutMax=[]  IntegratorOutMin=[]  IntegratorOutMax=[]  FilterOutMin=[]  FilterOutMax=[]  SumI1OutMin=[]  SumI1OutMax=[]  SumI2OutMin=[]  SumI2OutMax=[]  SumI3OutMin=[]  SumI3OutMax=[]  SumI4OutMin=[]  SumI4OutMax=[]  SumDOutMin=[]  SumDOutMax=[]  DifferentiatorOutMin=[]  DifferentiatorOutMax=[]  FilterDiffOutCoefMin=[]  FilterDiffOutCoefMax=[]  ReciprocalOutMin=[]  ReciprocalOutMax=[]  SumDenOutMin=[]  SumDenOutMax=[]  SumNumOutMin=[]  SumNumOutMax=[]  DivideOutMin=[]  DivideOutMax=[]  IntegratorContinuousStateAttributes=''  IntegratorStateMustResolveToSignalObject=off  IntegratorRTWStateStorageClass=Auto  FilterContinuousStateAttributes=''  FilterStateMustResolveToSignalObject=off  FilterRTWStateStorageClass=Auto  ParallelPVariant=InternalParameters  IdealPVariant=Disabled  IVariant=InternalParameters  DVariant=Disabled  IntegratorVariant=Continuous  SatVariant=Enabled  AWVariant=ContClampingParallel  PCopyVariant=Disabled  TRVariant=Disabled  FdbkBlocksVariant=Forward  IdealPFdbkVariant=Disabled  SatFdbkVariant=Disabled  DerivativeFilterVariant=Disabled  NVariant=Disabled  NCopyVariant=Disabled_SignalSpec  FilterICVariant=Disabled  IntegratorICVariant=InternalICs  ExternalResetVariant=Disabled  TRSumVariant=Passthrough  SumFdbkVariant=Disabled  SumVariant=Sum_PI
  Product : Product  Inputs=5
  Product1 : Product
  Switch : Switch  Criteria=u2 > Threshold
  Unit Delay1 : UnitDelay  SampleTime=-1
  vehSpd2motSpd : Gain  Gain=(msk_gear_ratio/msk_tire_radius)*9.549
  F_out_N : Outport
  wires:
  Gain/1 -> Braking Torque LUT/1
  Unit Delay1/1 -> vehSpd2motSpd/1, Add/1, Acceleration Torque LUT/1  "vehActSpd"
  Switch/1 -> F_out_N/1  "F_out"
  Braking Wheels/1 -> Product1/2  "T_brk"
  Acceleration Torque LUT/1 -> Product/5  "T_acc"
  Braking Torque LUT/1 -> Braking Wheels/1
  PID Controller/1 -> Switch/2, Acc_Pedal/1, Brk_Pedal/1  "PI_out_val"
  v_spdfdbk_mps/1 -> Unit Delay1/1
  v_spd_mps/1 -> Add/2
  Product1/1 -> Switch/3  "F_brk"
  Product/1 -> Switch/1  "F_acc"
  Add/1 -> PID Controller/1  "spd_error"
  Acc_Pedal/1 -> Acceleration Torque LUT/2
  Brk_Pedal/1 -> Gain/1
  Constant/1 -> Product/4
  Constant1/1 -> Product/3, Product1/1
  Constant2/1 -> Product/2
  Motor Continuous Torque LUT/1 -> Product/1
  vehSpd2motSpd/1 -> Motor Continuous Torque LUT/1  "motor_spd_rpm"

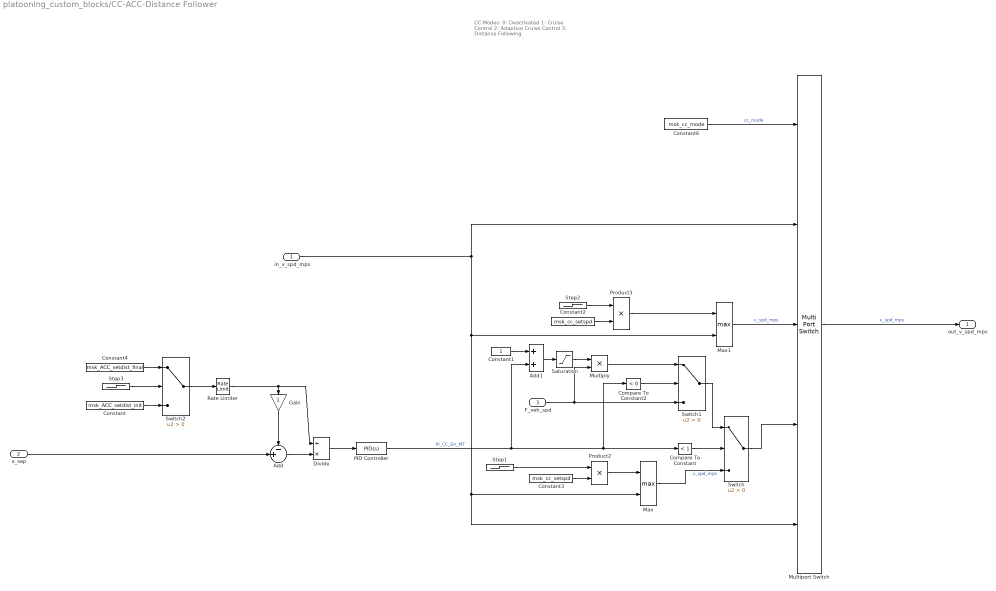
== system platooning_custom_blocks/CC-ACC-Distance Follower ==
  note: CC Modes:
      | 0: Deactivated
      | 1: Cruise Control
      | 2: Adaptive Cruise Control
      | 3: Distance Following
  in_v_spd_mps : Inport
  x_sep : Inport  Port=2
  F_veh_spd : Inport  Port=3
  Add : Sum  Inputs=-+|
  Add1 : Sum
  Compare To Constant : simulink/Logic and Bit Operations/Compare To Constant  relop=<  const=1  OutDataTypeStr=boolean
  Compare To Constant2 : simulink/Logic and Bit Operations/Compare To Constant  relop=<  const=0  OutDataTypeStr=boolean
  Constant : Constant  Value=msk_ACC_setdist_init
  Constant1 : Constant
  Constant2 : Constant  Value=msk_cc_setspd
  Constant3 : Constant  Value=msk_cc_setspd
  Constant4 : Constant  Value=msk_ACC_setdist_final
  Constant6 : Constant  Value=msk_cc_mode
  Divide : Product  Inputs=/*
  Gain : Gain
  Max : MinMax  Function=max  Inputs=2
  Max1 : MinMax  Function=max  Inputs=2
  Multiply : Product
  Multiport Switch : MultiPortSwitch  Inputs=4
  PID Controller : simulink/Continuous/PID Controller  Controller=PID  Form=Parallel  TimeDomain=Continuous-time  SampleTime=-1  IntegratorMethod=Forward Euler  FilterMethod=Forward Euler  ControllerParametersSource=internal  P=msk_ACC_Kp  I=msk_ACC_Ki  D=msk_ACC_Kd  UseFilter=on  N=100  TunerSelectOption=Transfer Function Based (PID Tuner App)  InitialConditionSource=internal  InitialConditionForIntegrator=0  InitialConditionForFilter=0  DifferentiatorICPrevScaledInput=0  ExternalReset=none  TrackingMode=off  Kt=1  LimitOutput=on  UpperSaturationLimit=1  LowerSaturationLimit=-1  LinearizeAsGain=on  AntiWindupMode=clamping  Kb=1  POutMin=[]  POutMax=[]  IOutMin=[]  IOutMax=[]  DOutMin=[]  DOutMax=[]  NOutMin=[]  NOutMax=[]  SumOutMin=[]  SumOutMax=[]  SaturationOutMin=[]  SaturationOutMax=[]  PParamMin=[]  PParamMax=[]  IParamMin=[]  IParamMax=[]  DParamMin=[]  DParamMax=[]  NParamMin=[]  NParamMax=[]  KbParamMin=[]  KbParamMax=[]  KtParamMin=[]  KtParamMax=[]  KbOutMin=[]  KbOutMax=[]  KtOutMin=[]  KtOutMax=[]  IntegratorOutMin=[]  IntegratorOutMax=[]  FilterOutMin=[]  FilterOutMax=[]  SumI1OutMin=[]  SumI1OutMax=[]  SumI2OutMin=[]  SumI2OutMax=[]  SumI3OutMin=[]  SumI3OutMax=[]  SumI4OutMin=[]  SumI4OutMax=[]  SumDOutMin=[]  SumDOutMax=[]  DifferentiatorOutMin=[]  DifferentiatorOutMax=[]  FilterDiffOutCoefMin=[]  FilterDiffOutCoefMax=[]  ReciprocalOutMin=[]  ReciprocalOutMax=[]  SumDenOutMin=[]  SumDenOutMax=[]  SumNumOutMin=[]  SumNumOutMax=[]  DivideOutMin=[]  DivideOutMax=[]  IntegratorContinuousStateAttributes=''  IntegratorStateMustResolveToSignalObject=off  IntegratorRTWStateStorageClass=Auto  FilterContinuousStateAttributes=''  FilterStateMustResolveToSignalObject=off  FilterRTWStateStorageClass=Auto  ParallelPVariant=InternalParameters  IdealPVariant=Disabled  IVariant=InternalParameters  DVariant=InternalParameters  IntegratorVariant=Continuous  SatVariant=Enabled  AWVariant=ContClampingParallel  PCopyVariant=Disabled  TRVariant=Disabled  FdbkBlocksVariant=Forward  IdealPFdbkVariant=Disabled  SatFdbkVariant=Disabled  DerivativeFilterVariant=ContFilter  NVariant=InternalParameters  NCopyVariant=Disabled  FilterICVariant=InternalICsFilter  IntegratorICVariant=InternalICs  ExternalResetVariant=Disabled  TRSumVariant=Passthrough  SumFdbkVariant=Disabled  SumVariant=Sum_PID
  Product2 : Product
  Product3 : Product
  Rate Limiter : RateLimiter  RisingSlewLimit=0.1  FallingSlewLimit=-0.1  SampleTimeMode=inherited  InitialCondition=msk_ACC_setdist_init
  Saturation : Saturate  UpperLimit=1  LowerLimit=0
  Step1 : Step  Time=msk_cc_time  SampleTime=0.1
  Step2 : Step  Time=msk_cc_time  SampleTime=0.1
  Step3 : Step  Time=msk_platoon_time  SampleTime=0.1
  Switch : Switch  Criteria=u2 > Threshold
  Switch1 : Switch  Criteria=u2 > Threshold
  Switch2 : Switch  Criteria=u2 > Threshold
  out_v_spd_mps : Outport
  wires:
  Switch2/1 -> Rate Limiter/1
  Step3/1 -> Switch2/2
  Constant4/1 -> Switch2/1
  Rate Limiter/1 -> Divide/1, Gain/1
  Multiply/1 -> Switch1/1
  Switch1/1 -> Switch/1
  Saturation/1 -> Multiply/1
  Add1/1 -> Saturation/1
  Compare To Constant2/1 -> Switch1/2
  Switch/1 -> Multiport Switch/4
  F_veh_spd/1 -> Switch1/3, Multiply/2
  Compare To Constant/1 -> Switch/2
  Constant/1 -> Switch2/3
  Divide/1 -> PID Controller/1
  Gain/1 -> Add/1
  Step2/1 -> Product3/1
  Product3/1 -> Max1/1
  Constant2/1 -> Product3/2
  Add/1 -> Divide/2
  Constant6/1 -> Multiport Switch/1  "cc_mode"
  Max1/1 -> Multiport Switch/3  "v_spd_mps"
  Multiport Switch/1 -> out_v_spd_mps/1  "v_spd_mps"
  x_sep/1 -> Add/2
  PID Controller/1 -> Add1/2, Compare To Constant2/1, Compare To Constant/1  "PI_CC_Err_MT"
  Constant1/1 -> Add1/1
  Constant3/1 -> Product2/2
  Step1/1 -> Product2/1
  Product2/1 -> Max/1
  in_v_spd_mps/1 -> Max/2, Multiport Switch/5, Max1/2, Multiport Switch/2
  Max/1 -> Switch/3  "v_spd_mps"

== system platooning_custom_blocks/Conventional Truck ==
  From_DTIL_BUS : Inport
  V_SPD : Inport  Port=2
  F_Dist_m : Inport  Port=3
  Cd : Inport  Port=4
  From_PCL : Inport  Port=5
  Init_Pos_m : Inport  Port=6
  2 DOF Longitudinal Dynamics Model - Force Input : $bdroot/2 DOF Longitudinal Dynamics Model - Force Input  msk_mass=CTModel.veh_mass_kg  msk_Af=CTModel.Af_m2  msk_Cd=CTModel.Cd_avg * ones([3 1])  msk_Cd_bpt=[5;10;15]  msk_r_tire=CTModel.ld_tire_rad_m  msk_v_init=init_veh_spd_mps  msk_roadType=Smooth Concrete  msk_rho_air=1.227  msk_tstep=sim_t_step
  Bus Creator1 : BusCreator  Inputs=4
  Bus Creator2 : BusCreator  Inputs=4
  Bus Creator3 : BusCreator  Inputs=4
  Bus Selector1 : BusSelector  OutputSignals=lead_grade_pct
  Conventional Post-Processing : Subsystem  mask{msk_fuel_init_liters=CTModel.fuelTankCap_L, msk_fuel_rho_kgpl=CTModel.fuelrho_kgpl, msk_fuel_lhv_kwhpkg=CTModel.fuelLHV_kwhpkg, msk_distwin=1000}
      mask prompts: msk_fuel_init_liters "Initial fuel level [L]:"; msk_fuel_rho_kgpl "Fuel density, rho [kg/L]:"; msk_fuel_lhv_kwhpkg "Fuel LHV [kWh/kg]:"; msk_distwin "Distance Window [m]:"
      mask DialogControl DescGroupVar Prompt: Conventional Vehicle Post-Processing
      mask DialogControl DescTextVar Prompt: This block computes the overall energy consumption and fuel consumption for a conventional vehicle.
      mask DialogControl ParameterGroupVar Prompt: Fuel/Fuel Tank Parameters
      mask DialogControl Container3 Prompt: Averaging Function Parameters
  Conventional Powertrain Energy Management System : Subsystem
  Conventional Powertrain Power Loss Model : Subsystem  mask{msk_tire_radius_m=CTModel.ld_tire_rad_m, msk_fd_ratio=CTModel.fd_ratio, msk_drv_eff=0.98, eng_pk_trq_vec=CTModel.peak_eng_trq_map, eng_pk_mtr_trq=CTModel.mtr_eng_trq_map, eng_spd_bpt=CTModel.peak_eng_trq_spd_bpt, msk_eng_fuel_map=CTModel.eng_fuel_map, msk_eng_trq_bpt=CTModel.eng_map_trq_bpt, msk_eng_spd_bpt=CTModel.eng_map_spd_bpt, msk_fuel_init_liters=CTModel.fuelTankCap_L, msk_rho_fuel_kgpL=CTModel.fuelrho_kgpl, msk_gear_rat_vec=CTModel.gear_ratios, msk_gear_eff_vec=CTModel.gear_eff, msk_init_gear=1, msk_P_aux_elec_load=CTModel.P_aux_elec, msk_P_aux_mech_load=CTModel.P_aux_mech, msk_load_frac=CTModel.P_aux_load_frac, msk_snr_P_aux=25, msk_alt_eff=0.90, msk_t_step=sim_t_step}
      mask prompts: msk_tire_radius_m "Loaded tire radius [m]:"; msk_fd_ratio "Final drive ratio [-]:"; msk_drv_eff "Driveline efficiency/100 [-]:"; eng_pk_trq_vec "Engine peak torque - propulsion [Nm]:"; eng_pk_mtr_trq "Engine peak torque - motoring [Nm]:"; eng_spd_bpt "Engine speed breakpoints [RPM]:"; msk_eng_fuel_map "Engine fuel map [g/s]:"; msk_eng_trq_bpt "Engine torque breakpoints [Nm]:"; msk_eng_spd_bpt "Engine speed breakpoints [RPM]:"; msk_fuel_init_liters "Initial fuel capacity [L]:"; msk_rho_fuel_kgpL "Fuel density [kg/L]:"; msk_gear_rat_vec "Gear ratio vector []:"; msk_gear_eff_vec "Gear efficiency vector []:"; msk_init_gear "Initial gear :"; msk_P_aux_elec_load "Auxiliary power load, electric [W]:"; msk_P_aux_mech_load "Auxiliary power load, mechanical [W]:"; msk_load_frac "Auxiliary load fraction [-]"; msk_snr_P_aux "Auxiliary load signal-to-noise ratio [-]:"; msk_alt_eff "Alternator efficiency/100 [-]:"; msk_t_step "Simulation time step [s]:"
      mask DialogControl DescGroupVar Prompt: Conventional Powertrain Power Loss Model
      mask DialogControl DescTextVar Prompt: Parameter settings for the powertrain components for the Conventional Powertrain Power Loss Model
      mask DialogControl Container10 Prompt: Vehicle Parameters
      mask DialogControl Container7 Prompt: Engine Parameters
      mask DialogControl Container12 Prompt: Torque Saturation Block Parameters
      mask DialogControl Container13 Prompt: Engine Fuel Map Parameters
      mask DialogControl Container14 Prompt: Fuel Parameters
      mask DialogControl Container9 Prompt: Transmission Parameters
      mask DialogControl Container4 Prompt: Auxiliary Load Parameters
      mask DialogControl Container11 Prompt: Simulation Parameters
  Conventional Truck Driver and Vehicle Acceleration Dynamics Model - Force Output : $bdroot/Conventional Truck Driver and  Vehicle Acceleration Dynamics Model  - Force Output  msk_Kp=0.1  msk_Ki=0.001  msk_t_step=sim_t_step  msk_gear_ratio_vec=CTModel.gear_ratios  msk_gearShft_UL=[3, 5, 9, 13, 17, 21, 25, 29, 33, 45]  msk_gearShft_LL=[0, 2, 4, 8, 12, 16, 20, 24, 28, 32]  msk_gearInit=1  msk_acc_trqmap=AccPdl_trqMap  msk_acc_spdbpt=AccPdl_spdbpt  msk_acc_pdlbpt=AccPdl_pdlbpt  msk_brk_trq=BrkPdl_brkTrq  msk_brk_pdlbpt=BrkPdl_pdlbpt  msk_mass=CTModel.veh_mass_kg  msk_damp_acc=800  msk_damp_brk=0.1  msk_fd_ratio=CTModel.fd_ratio  msk_tire_radius=CTModel.ld_tire_rad_m  msk_max_trq=max(CTModel.peak_eng_trq_map)  msk_brk_whl_num=18
  Rate Transition : RateTransition  OutPortSampleTime=sim_t_step
  Terminator : Terminator
  To_PCL : Outport
  wires:
  Cd/1 -> 2 DOF Longitudinal Dynamics Model - Force Input/4
  Init_Pos_m/1 -> Conventional Powertrain Power Loss Model/3(Init_Pos_m)
  Bus Creator3/1 -> Conventional Powertrain Power Loss Model/2(Power_data_bus)  "PowerDatBus"
  2 DOF Longitudinal Dynamics Model - Force Input/2 -> Bus Creator1/4  "vehAccOut"
  F_Dist_m/1 -> 2 DOF Longitudinal Dynamics Model - Force Input/3
  [gear_ratio] -> Bus Creator1/2
  2 DOF Longitudinal Dynamics Model - Force Input/7 -> Bus Creator3/1  "P_prop"
  2 DOF Longitudinal Dynamics Model - Force Input/5 -> Bus Creator2/3  "F_cr"
  2 DOF Longitudinal Dynamics Model - Force Input/8 -> Bus Creator3/2  "P_ar"
  V_SPD/1 -> Conventional Truck Driver and Vehicle Acceleration Dynamics Model - Force Output/3
  2 DOF Longitudinal Dynamics Model - Force Input/6 -> Bus Creator2/4  "F_rr"
  2 DOF Longitudinal Dynamics Model - Force Input/9 -> Bus Creator3/3  "P_cr"
  2 DOF Longitudinal Dynamics Model - Force Input/10 -> Bus Creator3/4  "P_rr"
  Bus Creator1/1 -> Conventional Powertrain Power Loss Model/1(Motion_data_bus)  "MotionDatBus"
  Bus Selector1/1 -> 2 DOF Longitudinal Dynamics Model - Force Input/2  "<lead_grade_pct>"
  Conventional Truck Driver and Vehicle Acceleration Dynamics Model - Force Output/3 -> Rate Transition/1  "F_cmd_out"
  Conventional Truck Driver and Vehicle Acceleration Dynamics Model - Force Output/2 -> [gear_ratio]
  2 DOF Longitudinal Dynamics Model - Force Input/1 -> Bus Creator1/3, Conventional Truck Driver and Vehicle Acceleration Dynamics Model - Force Output/1  "vehSpdOut"
  Conventional Powertrain Energy Management System/1(EMC_to_PropSys) -> Conventional Truck Driver and Vehicle Acceleration Dynamics Model - Force Output/2, Conventional Powertrain Power Loss Model/4(EM_control_bus)
  Bus Creator2/1 -> Terminator/1
  From_DTIL_BUS/1 -> Bus Selector1/1
  2 DOF Longitudinal Dynamics Model - Force Input/3 -> Bus Creator2/1  "F_prop"
  2 DOF Longitudinal Dynamics Model - Force Input/4 -> Bus Creator2/2  "F_ar"
  Rate Transition/1 -> 2 DOF Longitudinal Dynamics Model - Force Input/1
  Conventional Powertrain Power Loss Model/1(PropSys_to_EMC) -> Conventional Powertrain Energy Management System/1(PropSys_to_EMC), Conventional Post-Processing/1(PropSys_to_EMC)
  Conventional Post-Processing/1(To_PCL_BUS) -> To_PCL/1
  From_PCL/1 -> Conventional Powertrain Energy Management System/2(From_PCL_BUS)
  Conventional Truck Driver and Vehicle Acceleration Dynamics Model - Force Output/1 -> [gear_cmd]
  [gear_cmd] -> Bus Creator1/1
